simulink model "CarLightBehavior"  (R2024a)
settings: Solver=FixedStepAuto  StartTime=0.0  StopTime=10.0  FixedStep=0.1  RelTol=1e-3
settings Model: Creator=amir  LastModifiedBy=amir

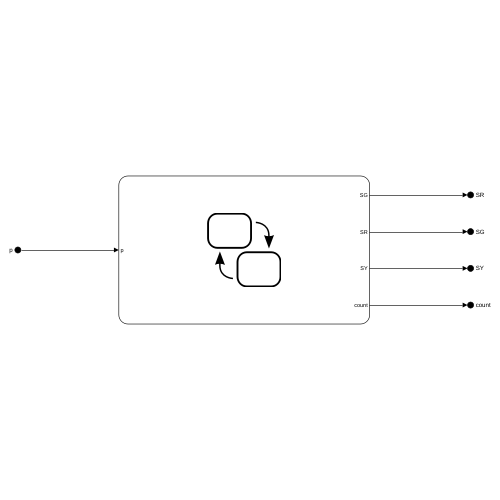
[thumbnail: Simulink's stored preview of the top-level diagram]
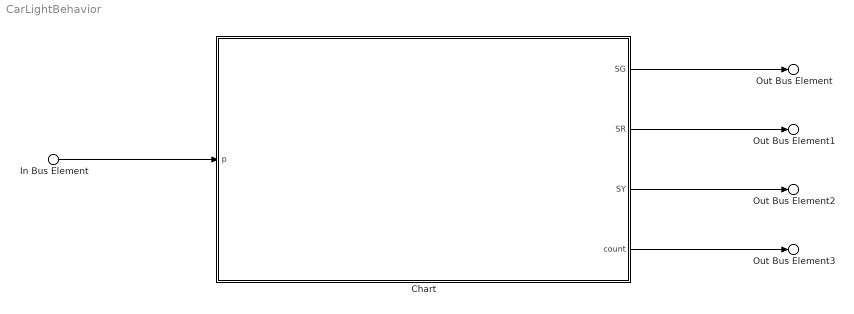
== system CarLightBehavior ==
  In Bus Element : Inport  PortName=p
  Chart : Stateflow chart  TreatAsAtomicUnit=on
  Out Bus Element : Outport  PortName=SR
  Out Bus Element1 : Outport  Port=2  PortName=SG
  Out Bus Element2 : Outport  Port=3  PortName=SY
  Out Bus Element3 : Outport  Port=4  PortName=count
  wires:
  Chart/1(SG) -> Out Bus Element/1
  Chart/2(SR) -> Out Bus Element1/1
  Chart/3(SY) -> Out Bus Element2/1
  Chart/4(count) -> Out Bus Element3/1
  In Bus Element/1 -> Chart/1(p)

== stateflow chart CarLightBehavior/Chart ==
  state Green
  state Red
  state Yellow
  state Pending
  Green -> Green [order 1] : [count<60]{count=count+1;}
  (default) -> Red : {count=0;}
  Red -> Green [order 1] : [count>=60]{SG=1; SR=0; count=0;}
  Green -> Yellow [order 2] : [p==1 && count<60]{SG=0;}
  Green -> Pending [order 3] : [p==1 && count>=60]{SG=0; SY=1; count=0;}
  Yellow -> Yellow [order 2] : {count=count+1}
  Red -> Red [order 2] : {count=count+1;}
  Pending -> Red [order 1] : [count>=5]{SR=1; count=0;}
  Yellow -> Pending [order 1] : [count>=60]{SY=1; count=0;}
  Pending -> Pending [order 2] : {count=count+1; SY=0}
  data: p input; SG output; SR output; SY output; count output
